simulink model "sf_electrohydraulic"  (Simulink 6.0)
settings: Solver=ode45  SolverMode=SingleTasking  StartTime=0.0  StopTime=2  FixedStep=0.2e-4  MaxStep=0.2e-3  RelTol=1e-3  AbsTol=1e-6
PreLoadFcn:
  | load sf_electrohydraulic
values from neighbouring files (symbols this model uses):
  m = sz(1)    [sf_edit_icon.m]
undefined symbols (not defined in the file or in its folder): A, Ao, Ap, balltravel, beta, Cv, dcmax, dcmin, dcnull, deltai, Fs0, gmax, gser, Ihold, Ipull, Ka, Ko, Ks, Ksp, Lsteel, Mp, mu0, N, Ps, R, Tpwm, Vd, Vs, Vz, xpmax, xpmin
libraries: simulink3 x1
settings Model: CovMetricSettings=dcmtr  Creator=The MathWorks Inc.  LastModifiedBy=batserve  ExtModeTrigMode=oneshot  ExtModeArmWhenConnect=off  ExtModeAutoUpdateStatusClock=off
settings DataIOCC: LimitDataPoints=off  SaveOutput=off  SaveTime=off
settings OptimizationCC: BooleanDataType=off
settings DebuggingCC: CheckExecutionContextPreStartOutputMsg=on  CheckExecutionContextRuntimeOutputMsg=on  SolverPrmCheckMsg=none  IntegerOverflowMsg=none
settings HardwareCC: TargetUnknown=on

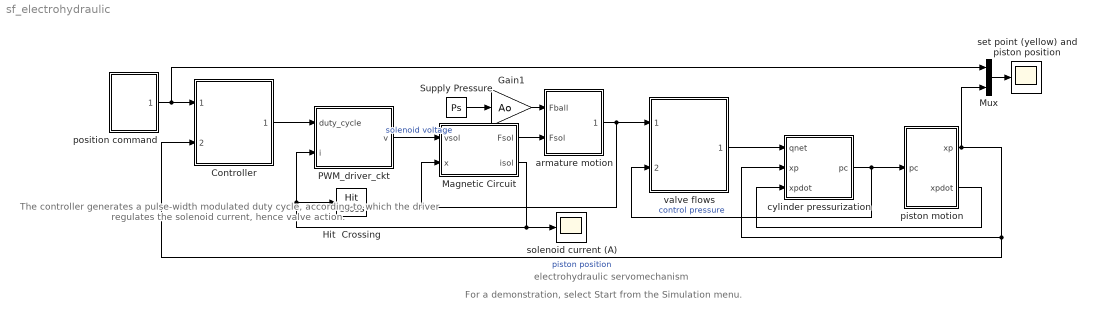
== system sf_electrohydraulic ==
  note: The controller generates a
      | pulse-width modulated duty
      | cycle, according to which the
      | driver regulates the solenoid
      | current, hence valve action.
  note: electrohydraulic servomechanism
  note: For a demonstration, select Start from the Simulation menu.
  Controller : Subsystem  PropExecContextAcrossSSBoundary=on
  Gain1 : Gain  Gain=Ao  SaturateOnIntegerOverflow=on
  Hit  Crossing : HitCross  HitCrossingOffset=[0, Ipull, (Ihold + deltai), (Ihold - deltai)]  ShowOutputPort=off
  Magnetic Circuit : Subsystem  PropExecContextAcrossSSBoundary=on
  Mux : Mux  Inputs=2
  PWM_driver_ckt : Stateflow chart  PropExecContextAcrossSSBoundary=on
  Supply Pressure : Constant  Value=Ps
  armature motion : Subsystem  PropExecContextAcrossSSBoundary=on
  cylinder pressurization : Subsystem  PropExecContextAcrossSSBoundary=on
  piston motion : Subsystem  PropExecContextAcrossSSBoundary=on
  position command : Subsystem  PropExecContextAcrossSSBoundary=on
  set point (yellow) and piston position : Scope
      settings: TickLabels=on  YMin=0.002  YMax=0.0175  DataFormat=Array  MaxDataPoints=5e4
  solenoid current (A) : Scope
      settings: TickLabels=on  TimeRange=0.02  YMin=-0.25  YMax=2.75  DataFormat=Array  MaxDataPoints=5e4
  valve flows : Subsystem  PropExecContextAcrossSSBoundary=on
  wires:
  Mux/1 -> set point (yellow) and piston position/1
  position command/1(set point) -> Controller/1(set point), Mux/1
  piston motion/2(xpdot) -> cylinder pressurization/3(xpdot)
  cylinder pressurization/1(pc) -> piston motion/1(pc), valve flows/2(control pressure)  "control pressure"
  valve flows/1(net flow) -> cylinder pressurization/1(qnet)
  piston motion/1(xp) -> Mux/2, cylinder pressurization/2(xp), Controller/2(feedback)  "piston position"
  armature motion/1(stroke) -> Magnetic Circuit/2(x), valve flows/1(armature position)
  Controller/1(duty cycle) -> PWM_driver_ckt/1(duty_cycle)
  PWM_driver_ckt/1(v) -> Magnetic Circuit/1(vsol)  "solenoid voltage"
  Magnetic Circuit/1(Fsol) -> armature motion/2(Fsol)
  Magnetic Circuit/2(isol) -> Hit  Crossing/1, PWM_driver_ckt/2(i), solenoid current (A)/1
  Gain1/1 -> armature motion/1(Fball)
  Supply Pressure/1 -> Gain1/1

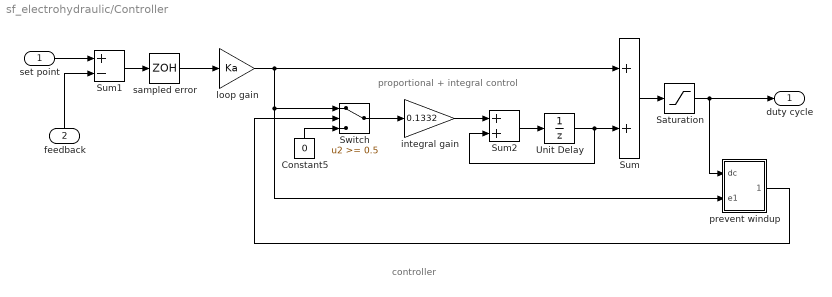
== system sf_electrohydraulic/Controller ==
  note: proportional + integral control
  note: controller
  set point : Inport  Port=1  LatchInput=off
  feedback : Inport  Orientation=up  Port=2  LatchInput=off
  Constant5 : Constant  Orientation=up  Value=0
  Saturation : Saturate  UpperLimit=dcmax  LowerLimit=dcmin
  Sum : Sum  SaturateOnIntegerOverflow=on  InputSameDT=on
  Sum1 : Sum  Inputs=+-  SaturateOnIntegerOverflow=on  InputSameDT=on
  Sum2 : Sum  SaturateOnIntegerOverflow=on  InputSameDT=on
  Switch : Switch  Threshold=0.5  SaturateOnIntegerOverflow=on  InputSameDT=on
  Unit Delay : UnitDelay  X0=dcnull  SampleTime=0.02
  integral gain : Gain  Gain=0.1332  SaturateOnIntegerOverflow=on
  loop gain : Gain  Gain=Ka  SaturateOnIntegerOverflow=on
  prevent windup : Subsystem  PropExecContextAcrossSSBoundary=on
  sampled error : ZeroOrderHold  SampleTime=0.02
  duty cycle : Outport  InitialOutput=0
  wires:
  sampled error/1 -> loop gain/1
  Sum1/1 -> sampled error/1
  Constant5/1 -> Switch/3
  Switch/1 -> integral gain/1
  prevent windup/1(nothold) -> Switch/2
  integral gain/1 -> Sum2/1
  Sum2/1 -> Unit Delay/1
  Unit Delay/1 -> Sum/2, Sum2/2
  set point/1 -> Sum1/1
  feedback/1 -> Sum1/2
  loop gain/1 -> prevent windup/2(e1), Switch/1, Sum/1
  Saturation/1 -> duty cycle/1, prevent windup/1(dc)
  Sum/1 -> Saturation/1

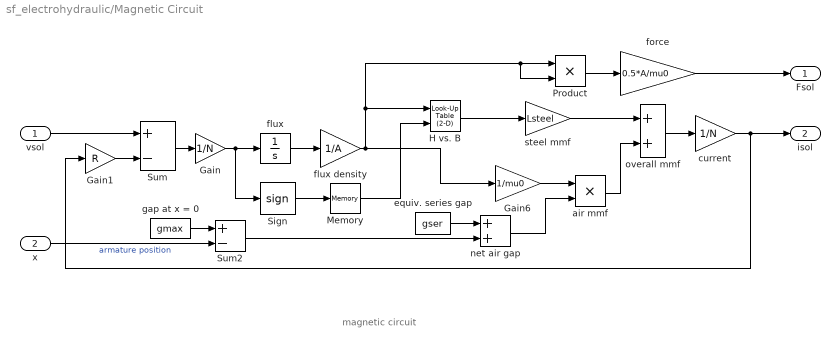
== system sf_electrohydraulic/Magnetic Circuit ==
  note: magnetic circuit
  vsol : Inport  Port=1  LatchInput=off
  x : Inport  Port=2  LatchInput=off
  Gain : Gain  Gain=1/N  SaturateOnIntegerOverflow=on
  Gain1 : Gain  Gain=R  SaturateOnIntegerOverflow=on
  Gain6 : Gain  Gain=1/mu0  SaturateOnIntegerOverflow=on
  H vs. B : simulink3/Functions & Tables/Look-Up Table (2-D)  x=Bvalues  y=[-1 1]  t=Hdata'
  Memory : Memory
  Product : Product  SaturateOnIntegerOverflow=on  RndMeth=Zero  InputSameDT=on
  Sign : Signum
  Sum : Sum  Inputs=+-  SaturateOnIntegerOverflow=on  InputSameDT=on
  Sum2 : Sum  Inputs=+-  SaturateOnIntegerOverflow=on  InputSameDT=on
  air mmf : Product  SaturateOnIntegerOverflow=on  RndMeth=Zero  InputSameDT=on
  current : Gain  Gain=1/N  SaturateOnIntegerOverflow=on
  equiv. series gap : Constant  Value=gser
  flux : Integrator  LowerSaturationLimit=0
  flux density : Gain  Gain=1/A  SaturateOnIntegerOverflow=on
  force : Gain  Gain=0.5*A/mu0  SaturateOnIntegerOverflow=on
  gap at x = 0 : Constant  Value=gmax
  net air gap : Sum  SaturateOnIntegerOverflow=on  InputSameDT=on
  overall mmf : Sum  SaturateOnIntegerOverflow=on  InputSameDT=on
  steel mmf : Gain  Gain=Lsteel  SaturateOnIntegerOverflow=on
  Fsol : Outport  InitialOutput=0
  isol : Outport  Port=2  InitialOutput=0
  wires:
  x/1 -> Sum2/2  "armature position"
  gap at x = 0/1 -> Sum2/1
  Sum2/1 -> net air gap/2
  equiv. series gap/1 -> net air gap/1
  Sum/1 -> Gain/1
  Gain1/1 -> Sum/2
  vsol/1 -> Sum/1
  net air gap/1 -> air mmf/2
  current/1 -> isol/1, Gain1/1
  flux density/1 -> H vs. B/1, Gain6/1, Product/2, Product/1
  overall mmf/1 -> current/1
  air mmf/1 -> overall mmf/2
  steel mmf/1 -> overall mmf/1
  H vs. B/1 -> steel mmf/1
  Gain6/1 -> air mmf/1
  Gain/1 -> flux/1, Sign/1
  Memory/1 -> H vs. B/2
  flux/1 -> flux density/1
  force/1 -> Fsol/1
  Product/1 -> force/1
  Sign/1 -> Memory/1

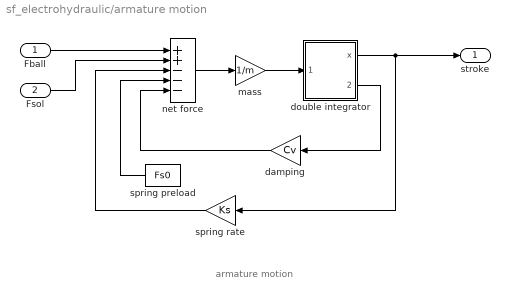
== system sf_electrohydraulic/armature motion ==
  note: armature motion
  Fball : Inport  Port=1  LatchInput=off
  Fsol : Inport  Port=2  LatchInput=off
  damping : Gain  Orientation=left  Gain=Cv  SaturateOnIntegerOverflow=on
  double integrator : Subsystem  PropExecContextAcrossSSBoundary=on
  mass : Gain  Gain=1/m  SaturateOnIntegerOverflow=on
  net force : Sum  Inputs=++---  SaturateOnIntegerOverflow=on  InputSameDT=on
  spring preload : Constant  Orientation=left  Value=Fs0
  spring rate : Gain  Orientation=left  Gain=Ks  SaturateOnIntegerOverflow=on
  stroke : Outport  InitialOutput=0
  wires:
  mass/1 -> double integrator/1(xdotdot)
  Fball/1 -> net force/1
  Fsol/1 -> net force/2
  spring rate/1 -> net force/3
  spring preload/1 -> net force/4
  damping/1 -> net force/5
  double integrator/2(xdot) -> damping/1
  net force/1 -> mass/1
  double integrator/1(x) -> spring rate/1, stroke/1

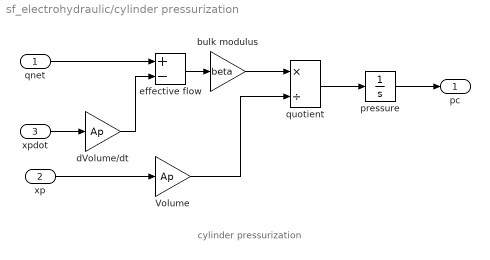
== system sf_electrohydraulic/cylinder pressurization ==
  note: cylinder pressurization
  qnet : Inport  Port=1  LatchInput=off
  xp : Inport  Port=2  LatchInput=off
  xpdot : Inport  Port=3  LatchInput=off
  Volume : Gain  Gain=Ap  SaturateOnIntegerOverflow=on
  bulk modulus : Gain  Gain=beta  SaturateOnIntegerOverflow=on
  dVolume/dt : Gain  Gain=Ap  SaturateOnIntegerOverflow=on
  effective flow : Sum  Inputs=+-  SaturateOnIntegerOverflow=on  InputSameDT=on
  pressure : Integrator  LimitOutput=on  LowerSaturationLimit=0
  quotient : Product  Inputs=*/  SaturateOnIntegerOverflow=on  RndMeth=Zero  InputSameDT=on
  pc : Outport  InitialOutput=0
  wires:
  xpdot/1 -> dVolume/dt/1
  dVolume/dt/1 -> effective flow/2
  bulk modulus/1 -> quotient/1
  quotient/1 -> pressure/1
  effective flow/1 -> bulk modulus/1
  xp/1 -> Volume/1
  Volume/1 -> quotient/2
  qnet/1 -> effective flow/1
  pressure/1 -> pc/1

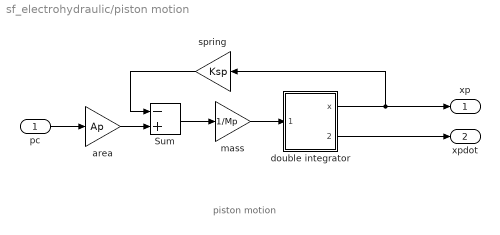
== system sf_electrohydraulic/piston motion ==
  note: piston motion
  pc : Inport  Port=1  LatchInput=off
  Sum : Sum  Inputs=-+  SaturateOnIntegerOverflow=on  InputSameDT=on
  area : Gain  Gain=Ap  SaturateOnIntegerOverflow=on
  double integrator : Subsystem  PropExecContextAcrossSSBoundary=on  mask{x0=xpmin, xmin=xpmin, xmax=xpmax, xdot0=0, xdotmin=-Inf, xdotmax=Inf}
      mask prompts: x0 "initial position"; xmin "minimum position"; xmax "maximum position"; xdot0 "initial velocity"; xdotmin "minimum velocity"; xdotmax "maximum velocity"
  mass : Gain  Gain=1/Mp  SaturateOnIntegerOverflow=on
  spring : Gain  Orientation=left  Gain=Ksp  SaturateOnIntegerOverflow=on
  xp : Outport  InitialOutput=0
  xpdot : Outport  Port=2  InitialOutput=0
  wires:
  pc/1 -> area/1
  double integrator/2(xdot) -> xpdot/1
  area/1 -> Sum/2
  Sum/1 -> mass/1
  spring/1 -> Sum/1
  mass/1 -> double integrator/1(xdotdot)
  double integrator/1(x) -> xp/1, spring/1

== system sf_electrohydraulic/position command ==
  Signal Generator : SignalGenerator  Amplitude=2e-3  Frequency=3
  Step : Step  Before=0.01  After=0.015  SampleTime=0
  Sum : Sum  SaturateOnIntegerOverflow=on  InputSameDT=on
  set point : Outport  InitialOutput=0
  wires:
  Step/1 -> Sum/1
  Signal Generator/1 -> Sum/2
  Sum/1 -> set point/1

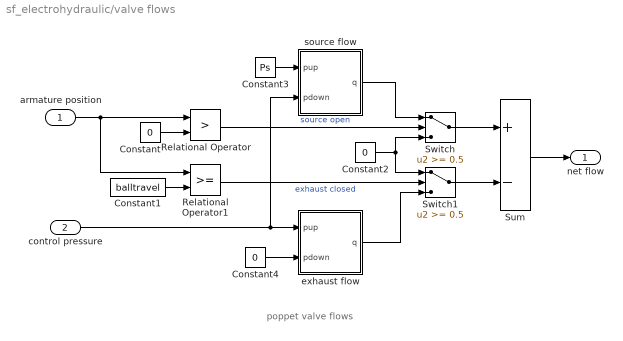
== system sf_electrohydraulic/valve flows ==
  note: poppet valve flows
  armature position : Inport  Port=1  LatchInput=off
  control pressure : Inport  Port=2  LatchInput=off
  Constant : Constant  Value=0
  Constant1 : Constant  Value=balltravel
  Constant2 : Constant  Value=0
  Constant3 : Constant  Value=Ps
  Constant4 : Constant  Value=0
  Relational Operator : RelationalOperator  Operator=>  InputSameDT=on
  Relational Operator1 : RelationalOperator  InputSameDT=on
  Sum : Sum  Inputs=+-  SaturateOnIntegerOverflow=on  InputSameDT=on
  Switch : Switch  Threshold=0.5  SaturateOnIntegerOverflow=on  InputSameDT=on
  Switch1 : Switch  Threshold=0.5  SaturateOnIntegerOverflow=on  InputSameDT=on
  exhaust flow : Subsystem  PropExecContextAcrossSSBoundary=on  mask(turbulent orifice flow){Ko=Ko, Ao=Ao}
      mask prompts: Ko "flow coefficient"; Ao "orifice area"
      mask Display: plot(-0.75,-1.25,0.75,1.25,[0 0],[1 -1],0.5*cos(-pi/4:.1:pi/4)-0.55, 0.5*sin(-pi/4:.1:pi/4),-0.5*cos(-pi/4:.1:pi/4)+0.55, 0.5*sin(-pi/4:.1:pi/4))
  source flow : Subsystem  PropExecContextAcrossSSBoundary=on  mask(turbulent orifice flow){Ko=Ko, Ao=Ao}
      mask prompts: Ko "flow coefficient"; Ao "orifice area"
      mask Display: plot(-0.75,-1.25,0.75,1.25,[0 0],[1 -1],0.5*cos(-pi/4:.1:pi/4)-0.55, 0.5*sin(-pi/4:.1:pi/4),-0.5*cos(-pi/4:.1:pi/4)+0.55, 0.5*sin(-pi/4:.1:pi/4))
  net flow : Outport  InitialOutput=0
  wires:
  Switch/1 -> Sum/1
  source flow/1(q) -> Switch/1
  Constant2/1 -> Switch/3, Switch1/1
  Constant/1 -> Relational Operator/2
  Constant3/1 -> source flow/1(pup)
  Relational Operator/1 -> Switch/2  "source open"
  Sum/1 -> net flow/1
  armature position/1 -> Relational Operator/1, Relational Operator1/1
  Constant4/1 -> exhaust flow/2(pdown)
  control pressure/1 -> exhaust flow/1(pup), source flow/2(pdown)
  Switch1/1 -> Sum/2
  Constant1/1 -> Relational Operator1/2
  Relational Operator1/1 -> Switch1/2  "exhaust closed"
  exhaust flow/1(q) -> Switch1/3

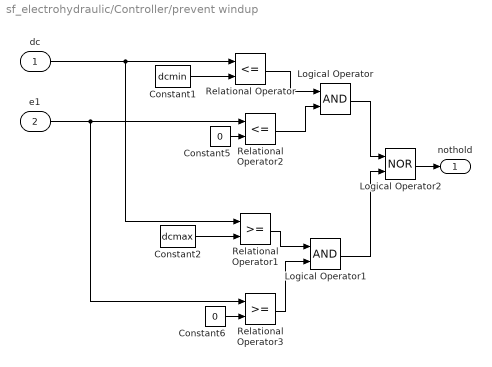
== system sf_electrohydraulic/Controller/prevent windup ==
  dc : Inport  Port=1  LatchInput=off
  e1 : Inport  Port=2  LatchInput=off
  Constant1 : Constant  Value=dcmin
  Constant2 : Constant  Value=dcmax
  Constant5 : Constant  Value=0
  Constant6 : Constant  Value=0
  Logical Operator : Logic
  Logical Operator1 : Logic
  Logical Operator2 : Logic  Operator=NOR
  Relational Operator : RelationalOperator  Operator=<=  InputSameDT=on
  Relational Operator1 : RelationalOperator  InputSameDT=on
  Relational Operator2 : RelationalOperator  Operator=<=  InputSameDT=on
  Relational Operator3 : RelationalOperator  InputSameDT=on
  nothold : Outport  InitialOutput=0
  wires:
  Logical Operator2/1 -> nothold/1
  Logical Operator1/1 -> Logical Operator2/2
  Logical Operator/1 -> Logical Operator2/1
  Relational Operator3/1 -> Logical Operator1/2
  Relational Operator1/1 -> Logical Operator1/1
  Constant6/1 -> Relational Operator3/2
  Constant5/1 -> Relational Operator2/2
  Relational Operator2/1 -> Logical Operator/2
  Constant2/1 -> Relational Operator1/2
  Relational Operator/1 -> Logical Operator/1
  Constant1/1 -> Relational Operator/2
  dc/1 -> Relational Operator/1, Relational Operator1/1
  e1/1 -> Relational Operator2/1, Relational Operator3/1

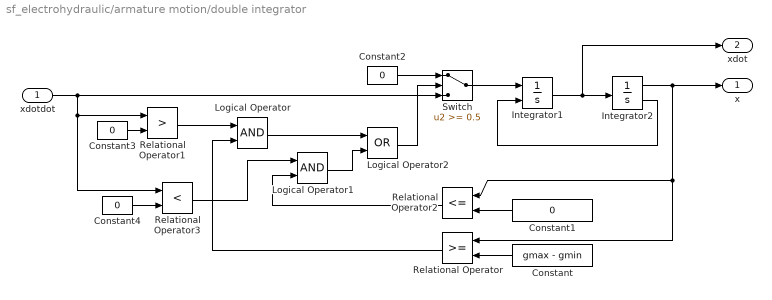
== system sf_electrohydraulic/armature motion/double integrator ==
  xdotdot : Inport  Port=1  LatchInput=off
  Constant : Constant  Orientation=left  Value=gmax - gmin
  Constant1 : Constant  Orientation=left  Value=0
  Constant2 : Constant  Value=0
  Constant3 : Constant  Value=0
  Constant4 : Constant  Value=0
  Integrator1 : Integrator  ExternalReset=rising  LowerSaturationLimit=Inf
  Integrator2 : Integrator  LimitOutput=on  UpperSaturationLimit=gmax - gmin  LowerSaturationLimit=0  ShowSaturationPort=on
  Logical Operator : Logic
  Logical Operator1 : Logic
  Logical Operator2 : Logic  Operator=OR
  Relational Operator : RelationalOperator  Orientation=left  InputSameDT=on
  Relational Operator1 : RelationalOperator  Operator=>  InputSameDT=on
  Relational Operator2 : RelationalOperator  Orientation=left  Operator=<=  InputSameDT=on
  Relational Operator3 : RelationalOperator  Operator=<  InputSameDT=on
  Switch : Switch  Threshold=0.5  SaturateOnIntegerOverflow=on  InputSameDT=on
  x : Outport  InitialOutput=0
  xdot : Outport  Port=2  InitialOutput=0
  wires:
  Integrator1/1 -> xdot/1, Integrator2/1
  Constant/1 -> Relational Operator/2
  Relational Operator/1 -> Logical Operator/2
  Relational Operator2/1 -> Logical Operator1/2
  Constant1/1 -> Relational Operator2/2
  xdotdot/1 -> Switch/3, Relational Operator1/1, Relational Operator3/1
  Constant3/1 -> Relational Operator1/2
  Relational Operator1/1 -> Logical Operator/1
  Constant4/1 -> Relational Operator3/2
  Relational Operator3/1 -> Logical Operator1/1
  Logical Operator/1 -> Logical Operator2/1
  Logical Operator1/1 -> Logical Operator2/2
  Constant2/1 -> Switch/1
  Logical Operator2/1 -> Switch/2
  Integrator2/2 -> Integrator1/2
  Switch/1 -> Integrator1/1
  Integrator2/1 -> x/1, Relational Operator/1, Relational Operator2/1

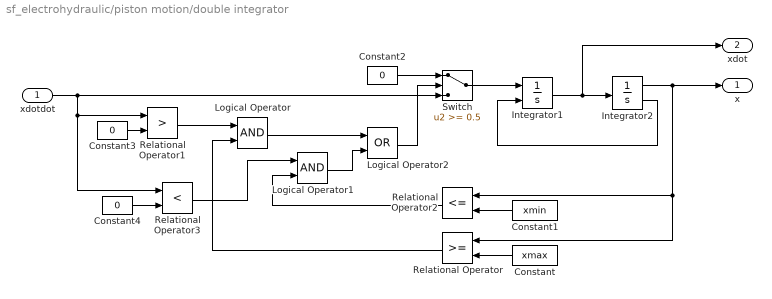
== system sf_electrohydraulic/piston motion/double integrator ==
  xdotdot : Inport  Port=1  LatchInput=off
  Constant : Constant  Orientation=left  Value=xmax
  Constant1 : Constant  Orientation=left  Value=xmin
  Constant2 : Constant  Value=0
  Constant3 : Constant  Value=0
  Constant4 : Constant  Value=0
  Integrator1 : Integrator  ExternalReset=rising  InitialCondition=xdot0  UpperSaturationLimit=xdotmax  LowerSaturationLimit=xdotmin
  Integrator2 : Integrator  InitialCondition=x0  LimitOutput=on  UpperSaturationLimit=xmax  LowerSaturationLimit=xmin  ShowSaturationPort=on
  Logical Operator : Logic
  Logical Operator1 : Logic
  Logical Operator2 : Logic  Operator=OR
  Relational Operator : RelationalOperator  Orientation=left  InputSameDT=on
  Relational Operator1 : RelationalOperator  Operator=>  InputSameDT=on
  Relational Operator2 : RelationalOperator  Orientation=left  Operator=<=  InputSameDT=on
  Relational Operator3 : RelationalOperator  Operator=<  InputSameDT=on
  Switch : Switch  Threshold=0.5  SaturateOnIntegerOverflow=on  InputSameDT=on
  x : Outport  InitialOutput=0
  xdot : Outport  Port=2  InitialOutput=0
  wires:
  Integrator2/1 -> Relational Operator2/1, Relational Operator/1, x/1
  Switch/1 -> Integrator1/1
  Integrator2/2 -> Integrator1/2
  Logical Operator2/1 -> Switch/2
  Constant2/1 -> Switch/1
  Logical Operator1/1 -> Logical Operator2/2
  Logical Operator/1 -> Logical Operator2/1
  Relational Operator3/1 -> Logical Operator1/1
  Constant4/1 -> Relational Operator3/2
  Relational Operator1/1 -> Logical Operator/1
  Constant3/1 -> Relational Operator1/2
  xdotdot/1 -> Relational Operator3/1, Relational Operator1/1, Switch/3
  Constant1/1 -> Relational Operator2/2
  Relational Operator2/1 -> Logical Operator1/2
  Relational Operator/1 -> Logical Operator/2
  Constant/1 -> Relational Operator/2
  Integrator1/1 -> Integrator2/1, xdot/1

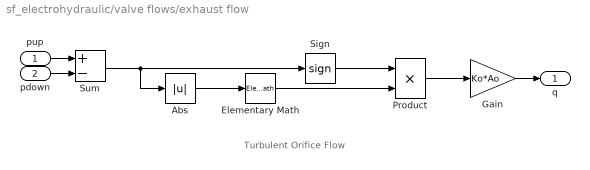
== system sf_electrohydraulic/valve flows/exhaust flow ==
  note: Turbulent Orifice Flow
  pup : Inport  Port=1  LatchInput=off
  pdown : Inport  Port=2  LatchInput=off
  Abs : Abs  SaturateOnIntegerOverflow=on
  Elementary Math : ElementaryMath  Operator=sqrt
  Gain : Gain  Gain=Ko*Ao  SaturateOnIntegerOverflow=on
  Product : Product  SaturateOnIntegerOverflow=on  RndMeth=Zero  InputSameDT=on
  Sign : Signum
  Sum : Sum  Inputs=+-  SaturateOnIntegerOverflow=on  InputSameDT=on
  q : Outport  InitialOutput=0
  wires:
  Gain/1 -> q/1
  pdown/1 -> Sum/2
  pup/1 -> Sum/1
  Sum/1 -> Abs/1, Sign/1
  Product/1 -> Gain/1
  Abs/1 -> Elementary Math/1
  Elementary Math/1 -> Product/2
  Sign/1 -> Product/1

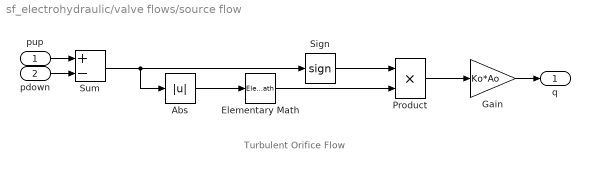
== system sf_electrohydraulic/valve flows/source flow ==
  note: Turbulent Orifice Flow
  pup : Inport  Port=1  LatchInput=off
  pdown : Inport  Port=2  LatchInput=off
  Abs : Abs  SaturateOnIntegerOverflow=on
  Elementary Math : ElementaryMath  Operator=sqrt
  Gain : Gain  Gain=Ko*Ao  SaturateOnIntegerOverflow=on
  Product : Product  SaturateOnIntegerOverflow=on  RndMeth=Zero  InputSameDT=on
  Sign : Signum
  Sum : Sum  Inputs=+-  SaturateOnIntegerOverflow=on  InputSameDT=on
  q : Outport  InitialOutput=0
  wires:
  Sign/1 -> Product/1
  Elementary Math/1 -> Product/2
  Abs/1 -> Elementary Math/1
  Product/1 -> Gain/1
  Sum/1 -> Sign/1, Abs/1
  pup/1 -> Sum/1
  pdown/1 -> Sum/2
  Gain/1 -> q/1

== stateflow chart PWM_driver_ckt ==
  settings: description=|
      | The objective is to direct fluid from supply to control when the duty
      |  cycle is high, and from control to exhaust when low.  The solenoid
      | is energized for the high portion.  This requires a current which is
      | initially large to pull the solenoid armature into its energized position,
      | and then somewhat lower to hold it in for the remainder of the high
      | phase of each PWM pulse.
  state energize_solenoid
    state pull_in_current
      entry : v = Vs;
    state regulate_hold_current
      state freewheel
        entry: v = -(i > 0)*Vd;
        during: v = -(i > 0)*Vd;
      state hold/
        entry : v = Vs;
      (default) -> freewheel
      freewheel -> hold : [ i <= Ihold - deltai ]
      hold -> freewheel : [ i >= Ihold + deltai ]
    (default) -> pull_in_current
    pull_in_current -> regulate_hold_current : [ i >= Ipull ]
  state solenoid_off
    entry : v = -(i > 0)*Vz;
    during: v = -(i > 0)*Vz;
  (default) -> (junction 9) : { ton = 0; }
  (junction 9) -> energize_solenoid : { toff = ton + duty_cycle*Tpwm/100; }
  solenoid_off -> (junction 9) : [ t >= ton ]
  energize_solenoid -> solenoid_off : [ t > toff ]
      | { ton += Tpwm;}
  data: v output double; duty_cycle input double [0..100]; ton local double; toff local double; Tpwm parameter double; Ipull parameter double; Ihold parameter double; deltai parameter double; Vs parameter double; Vz parameter double; Vd parameter double; i input double
  data v settings: units=volts  description=applied solenoid voltage
  data duty_cycle settings: units=%  description=pulse-width modulation duty cycle
  data ton settings: units=seconds  description=absolute time at the beginning of each PWM cycle
  data toff settings: units=seconds  description=absolute time at which the current PWM cycle switches off
  data Tpwm settings: units=seconds  description=pulse-width modulation period
  data Ipull settings: units=A  description=solenoid pull-in current, generates maximum force to move armature
  data Ihold settings: units=A  description=solenoid hold current (maintain armature in energized position)
  data deltai settings: units=A  description=switch-mode current regulation error width
  data Vs settings: units=volts  description=power supply voltage
  data Vz settings: units=volts  description=zener diode voltage
  data Vd settings: units=volts  description=freewheel diode forward voltage drop
  data i settings: units=A  description=solenoid current
